simulink model "Manuf30_M8"  (R2023a)
settings: Solver=FixedStepAuto  StartTime=0.0  StopTime=720  FixedStep=1  RelTol=1e-3
model workspace (MAT data in the model file):
  EPdefault = 5
  EPmax = 5
  FRm = 120
  IPdefault = 5
libraries: simulink x25
(part 1 of 2)
settings Model: PacingRate=63  Creator=Boris Petrenj  LastModifiedBy=bramb
settings OptimizationCC: DefaultParameterBehavior=Inlined  EnhancedBackFolding=on  PassReuseOutputArgsAs=Individual arguments  ZeroExternalMemoryAtStartup=off  ZeroInternalMemoryAtStartup=off  OptimizeBlockOrder=speed  DifferentSizesBufferReuse=on  OptimizationCustomize=off  EfficientTunableParamExpr=on
settings DebuggingCC: ParameterTunabilityLossMsg=error  UnconnectedInputMsg=warning  UnconnectedOutputMsg=warning  UnconnectedLineMsg=warning  UnderSpecifiedDimensionMsg=warning
settings HardwareCC: TargetBitPerPointer=64  TargetBitPerSizeT=64  TargetBitPerPtrDiffT=64  TargetLongLongMode=on  TargetIntDivRoundTo=Zero  TargetEndianess=LittleEndian  TargetWordSize=64  TargetHWDeviceType=MATLAB Host  ProdEqTarget=off
settings ModelReferenceCC: EnableRefExpFcnMdlSchedulingChecks=on
settings SFSimCC: MATLABDynamicMemAlloc=off
settings RTWCC: Description=Embedded Coder  SystemTargetFile=ert.tlc  TemplateMakefile=ert_default_tmf  RTWVerbose=off  DLArmComputeVersion=19.05
settings CodeAppCC: ForceParamTrailComments=on  IgnoreCustomStorageClasses=off  OperatorAnnotations=on  SimulinkDataObjDesc=on  SFDataObjDesc=on  InsertBlockDesc=on
settings ERTTargetCC: GenerateSampleERTMain=on  SupportContinuousTime=on  InlinedParameterPlacement=NonHierarchical  ERTCustomFileTemplate=example_file_process.tlc

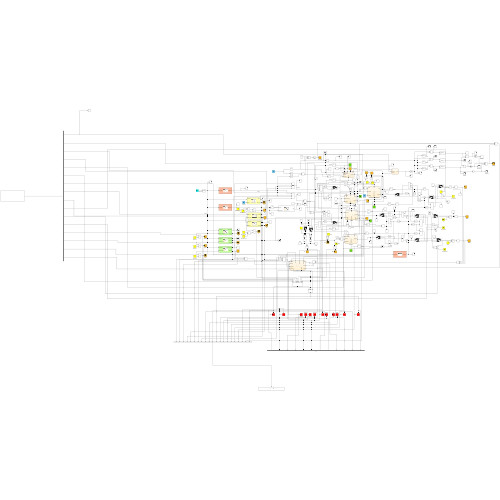
[thumbnail: Simulink's stored preview of the top-level diagram]
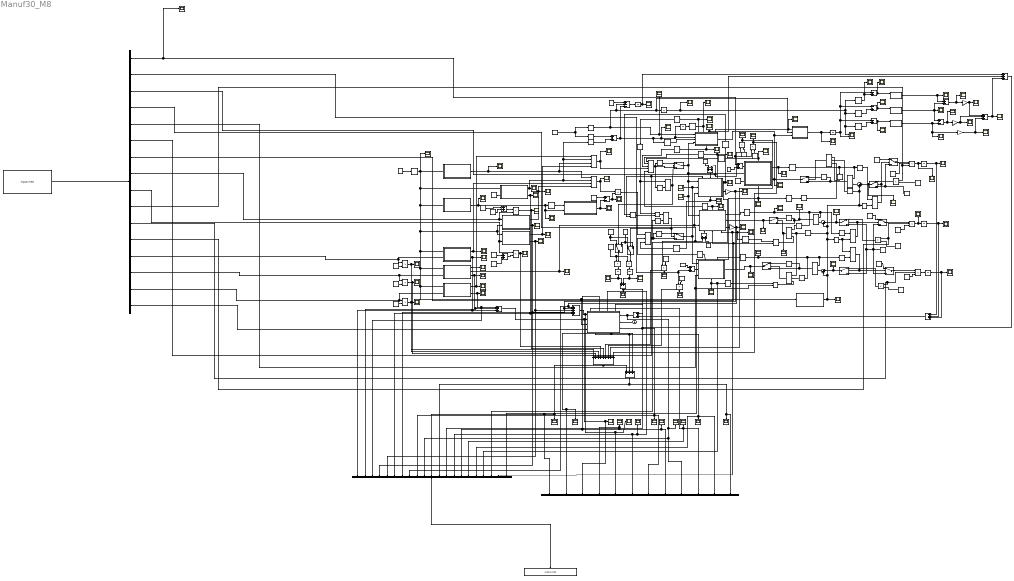
== system Manuf30_M8 ==
  AB : Scope
  AB deployment : Constant  Value=0.05
  ABackup price : Constant  Value=0.075
  AED : Scope
  Add : Sum  Inputs=+-
  Add{1,5..9,18..20} (9 alike) : Sum
  Add10 : Sum  Inputs=+-
  Add11 : Sum  Inputs=+-
  Add{12,14,16..17,22} (5 alike) : Sum  Inputs=+++
  Add13 : Sum  Inputs=+--
  Add15 : Sum  Inputs=+++++
  Add2 : Sum  Inputs=-+
  Add21 : Sum  Inputs=+++++++++
  Add3 : Sum  Inputs=-+
  Add4 : Sum  Inputs=-+
  BCI : Scope
  CancelledOrd : Scope
  Chart : Stateflow chart  TreatAsAtomicUnit=on
      settings: PortSchema="{\"entries\":[{\"content\":{\"sides\":[{\"content\":{\"connectorIds\":[\"In4\",\"In6\",\"In3\",\"In1\"]},\"type\":\"ConnectorPlacement.EquallySpacedRectSide\",\"uuid\":\"11f0d52a-88fc-4be5-bdc7-a55aa2612482\"},{\"content\":{\"connectorIds\":[\"In5\"],\"side\":\"RIGHT\"},\"type\":\"ConnectorPlacement.EquallySpacedRectSide\",\"uuid\":\"6f764515-397a-44dd-a2e9-3187fcbf9d3b\"},{\"content\":{\"connectorIds\":[\"Out3\",\"In2\",\"Out2\",\"In7\"],\"side\":\"TOP\"},\"type\":\"ConnectorPlacement.EquallySpacedRectSide\",\"uuid\":\"b2e58044-1c1f-45c5-a6c7-94a0948bfd55\"},{\"content\":{\"connectorIds\":[\"Out1\"],\"side\":\"BOTTOM\"},\"type\":\"ConnectorPlacement.EquallySpacedRectSide\",\"uuid\":\"446d024b-4857-45c6-b7aa-d3981b2b5c40\"}]},\"type\":\"ConnectorPlacement.EquallySpacedConnector\",\"uuid\":\"b78e99a1-1936-4240-9e27-63b28b547cdb\"}],\"packageUris\":[\"http://schema.mathworks.com/mf0/Connector/R2020b\"],\"version\":\"1.0\"}"
  Chart1 : Stateflow chart  TreatAsAtomicUnit=on
      settings: PortSchema="{\"entries\":[{\"content\":{\"sides\":[{\"content\":{\"connectorIds\":[\"In3\",\"In2\",\"In4\",\"In5\"]},\"type\":\"ConnectorPlacement.EquallySpacedRectSide\",\"uuid\":\"378523c1-40c5-4401-902f-aeb832ff0c9f\"},{\"content\":{\"connectorIds\":[\"In6\",\"In7\",\"In1\"],\"side\":\"RIGHT\"},\"type\":\"ConnectorPlacement.EquallySpacedRectSide\",\"uuid\":\"7940ff85-ee40-44d5-9690-9128d9333e88\"},{\"content\":{\"connectorIds\":[\"Out3\",\"Out5\",\"Out6\",\"Out4\"],\"side\":\"TOP\"},\"type\":\"ConnectorPlacement.EquallySpacedRectSide\",\"uuid\":\"ed54a4f9-7485-4487-a378-6fa31cb94842\"},{\"content\":{\"connectorIds\":[\"Out1\",\"Out2\"],\"side\":\"BOTTOM\"},\"type\":\"ConnectorPlacement.EquallySpacedRectSide\",\"uuid\":\"59aa636e-9062-4d7b-b9aa-b7c99c05c2d5\"}]},\"type\":\"ConnectorPlacement.EquallySpacedConnector\",\"uuid\":\"5563ec8e-56bc-49dd-8f68-3b08d3fc6c7f\"}],\"packageUris\":[\"http://schema.mathworks.com/mf0/Connector/R2020b\"],\"version\":\"1.0\"}"
  Chart2 : Stateflow chart  TreatAsAtomicUnit=on
      settings: PortSchema="{\"entries\":[{\"content\":{\"sides\":[{\"content\":{\"connectorIds\":[\"Out1\",\"In2\",\"In1\"]},\"type\":\"ConnectorPlacement.EquallySpacedRectSide\",\"uuid\":\"1d54177f-2d9d-4f9f-bcdb-576a16328a05\"},{\"content\":{\"connectorIds\":[\"Out2\"],\"side\":\"RIGHT\"},\"type\":\"ConnectorPlacement.EquallySpacedRectSide\",\"uuid\":\"203a6c5b-a59e-424a-95d4-58501034805f\"},{\"content\":{\"connectorIds\":[],\"side\":\"TOP\"},\"type\":\"ConnectorPlacement.EquallySpacedRectSide\",\"uuid\":\"eef511bd-9515-4db3-88d2-ce1a818e3fa2\"}]},\"type\":\"ConnectorPlacement.EquallySpacedConnector\",\"uuid\":\"79254a1d-868f-4542-aa12-bb7c48326cb6\"}],\"packageUris\":[\"http://schema.mathworks.com/mf0/Connector/R2020b\"],\"version\":\"1.0\"}"
  Clock : Clock
  Compare To Constant{,2..3,9} (4 alike) : simulink/Logic and Bit Operations/Compare To Constant  relop=>  const=0.9  OutDataTypeStr=boolean
  Compare To Constant1 : simulink/Logic and Bit Operations/Compare To Constant  relop=>  const=1  OutDataTypeStr=boolean
  Compare To Constant10 : simulink/Logic and Bit Operations/Compare To Constant  relop=>=  const=1.7  OutDataTypeStr=boolean
  Compare To Constant11 : simulink/Logic and Bit Operations/Compare To Constant  relop=>  const=1  OutDataTypeStr=boolean
  Compare To Constant12 : simulink/Logic and Bit Operations/Compare To Constant  relop=<  const=0.9  OutDataTypeStr=boolean
  Compare To Constant13 : simulink/Logic and Bit Operations/Compare To Constant  relop=>  const=0  OutDataTypeStr=boolean
  Compare To Constant4 : simulink/Logic and Bit Operations/Compare To Constant  relop=<  const=0.9  OutDataTypeStr=boolean
  Compare To Constant5 : simulink/Logic and Bit Operations/Compare To Constant  relop=>=  const=1.7  OutDataTypeStr=boolean
  Compare To Constant6 : simulink/Logic and Bit Operations/Compare To Constant  relop=>=  const=1.7  OutDataTypeStr=boolean
  Compare To Constant7 : simulink/Logic and Bit Operations/Compare To Constant  relop=>  const=0  OutDataTypeStr=boolean
  Compare To Constant8 : simulink/Logic and Bit Operations/Compare To Constant  relop=>  const=0  OutDataTypeStr=boolean
  Const : Constant  Value=0
  Const1 : Constant  Value=0
  Const{2..3,5..6} (4 alike) : Constant
  Const4 : Constant  Value=0
  Constant : Constant
  Constant11 : Constant  Value=8.5
  Constant2 : Constant
  Constant3 : Constant
  Delay : Delay  DelayLength=30  DelayLengthUpperLimit=5  InitialCondition=1  SampleTime=1
  Delay{1..3,5,7..8} (6 alike) : Delay  DelayLength=1  DelayLengthUpperLimit=5  InitialCondition=3  SampleTime=1
  Delay10 : Delay  DelayLength=1  DelayLengthUpperLimit=5  InitialCondition=IPdefault  SampleTime=1
  Delay{4,6,9,11..12,17} (6 alike) : Delay  DelayLength=1  DelayLengthUpperLimit=5  InitialCondition=1  SampleTime=1
  Delay13 : Delay  DelayLength=1  DelayLengthUpperLimit=5  InitialCondition=EPdefault  SampleTime=1
  Delay14 : Delay  DelayLength=60  DelayLengthUpperLimit=5  InitialCondition=0  SampleTime=1
  Delay15 : Delay  DelayLength=90  DelayLengthUpperLimit=5  InitialCondition=0  SampleTime=1
  Delay16 : Delay  DelayLength=30  DelayLengthUpperLimit=5  InitialCondition=0  SampleTime=1
  Delay18 : Delay  DelayLength=20  DelayLengthUpperLimit=5  InitialCondition=0.5  SampleTime=1
  Delay19 : Delay  DelayLength=100  DelayLengthUpperLimit=5  InitialCondition=0  SampleTime=1
  Delay20 : Delay  DelayLength=20  DelayLengthUpperLimit=5  InitialCondition=0  SampleTime=1
  Delay30 : Scope
  Delay60 : Scope
  Delay90 : Scope
  Demux : Demux  Outputs=16
  EP max : Constant  Value=10
  EPC : Constant  Value=0.01
  EPLoss : Scope
  EPS : Scope
  External : Stateflow chart  TreatAsAtomicUnit=on
      settings: PortSchema="{\"entries\":[{\"content\":{\"sides\":[{\"content\":{\"connectorIds\":[\"In1\",\"In4\"]},\"type\":\"ConnectorPlacement.EquallySpacedRectSide\",\"uuid\":\"f271faee-6a60-479d-a866-8a5439de7add\"},{\"content\":{\"connectorIds\":[\"Out1\",\"In5\",\"Out4\"],\"side\":\"RIGHT\"},\"type\":\"ConnectorPlacement.EquallySpacedRectSide\",\"uuid\":\"e4108372-e6fe-4c4b-a7e6-7abfa79efbb7\"},{\"content\":{\"connectorIds\":[\"Out2\"],\"side\":\"TOP\"},\"type\":\"ConnectorPlacement.EquallySpacedRectSide\",\"uuid\":\"57ee2673-3adc-41fc-b7cf-33ada2fd2761\"},{\"content\":{\"connectorIds\":[\"In2\",\"In3\",\"Out3\"],\"side\":\"BOTTOM\"},\"type\":\"ConnectorPlacement.EquallySpacedRectSide\",\"uuid\":\"ef56ac79-8641-40f7-a011-edb5fa111627\"}]},\"type\":\"ConnectorPlacement.EquallySpacedConnector\",\"uuid\":\"67aaf845-721f-4bae-9783-ff666cd7a7bd\"}],\"packageUris\":[\"http://schema.mathworks.com/mf0/Connector/R2020b\"],\"version\":\"1.0\"}"
  FINAL : Scope
  "FPC " : Constant  Value=0.012
  FPS : Scope
  FPdefault : Constant
  FPmax : Constant  Value=10
  Finished Products Warehouse : Stateflow chart  TreatAsAtomicUnit=on
      settings: PortSchema="{\"entries\":[{\"content\":{\"sides\":[{\"content\":{\"connectorIds\":[\"In3\",\"In2\",\"In1\"]},\"type\":\"ConnectorPlacement.EquallySpacedRectSide\",\"uuid\":\"a927ef52-d91a-4dcc-84e0-b91b0cab93cc\"},{\"content\":{\"connectorIds\":[\"Out2\",\"In4\"],\"side\":\"RIGHT\"},\"type\":\"ConnectorPlacement.EquallySpacedRectSide\",\"uuid\":\"3748cd02-f2f9-44a2-8c75-23a4abadb7cf\"},{\"content\":{\"connectorIds\":[\"Out1\"],\"side\":\"TOP\"},\"type\":\"ConnectorPlacement.EquallySpacedRectSide\",\"uuid\":\"31dbc187-02a7-4af9-af69-01f7c7d572fd\"},{\"content\":{\"connectorIds\":[\"Out3\"],\"side\":\"BOTTOM\"},\"type\":\"ConnectorPlacement.EquallySpacedRectSide\",\"uuid\":\"61372254-f33a-42e5-a460-357783406dca\"}]},\"type\":\"ConnectorPlacement.EquallySpacedConnector\",\"uuid\":\"01135270-3585-4456-b5cd-d6a08ddd9ae5\"}],\"packageUris\":[\"http://schema.mathworks.com/mf0/Connector/R2020b\"],\"version\":\"1.0\"}"
  From File : FromFile  FileName=input.mat  SampleTime=0
  Gain : Gain  Gain=0.8
  Gain1 : Gain  Gain=0.5
  Gain2 : Gain  Gain=0.2
  Gain4 : Gain  Gain=0.2
  Gain5 : Gain  Gain=0.4
  IPC : Constant  Value=0.01
  IPLoss : Scope
  IPS : Scope
  IPmax : Constant  Value=10
  IT backup : Constant  Value=0
  ITC : Constant  Value=0.002
  ITC1 : Constant  Value=0.002
  ITD : Scope
  InEPC : Scope
  InRMC : Scope
  Integrator{,1..8} (9 alike) : Integrator  ZeroCross=off
  Internal : Stateflow chart  TreatAsAtomicUnit=on
      settings: PortSchema="{\"entries\":[{\"content\":{\"sides\":[{\"content\":{\"connectorIds\":[\"In1\",\"In4\",\"In5\"]},\"type\":\"ConnectorPlacement.EquallySpacedRectSide\",\"uuid\":\"bafe3ab1-f241-4393-bddb-ef475e1fdd49\"},{\"content\":{\"connectorIds\":[\"Out4\",\"Out1\"],\"side\":\"RIGHT\"},\"type\":\"ConnectorPlacement.EquallySpacedRectSide\",\"uuid\":\"094e9ebe-ff1f-4efe-a044-3eef12cc294d\"},{\"content\":{\"connectorIds\":[\"In3\",\"In2\",\"Out2\"],\"side\":\"TOP\"},\"type\":\"ConnectorPlacement.EquallySpacedRectSide\",\"uuid\":\"3b7b6677-6a8b-48f7-ba0f-1ece0b251949\"},{\"content\":{\"connectorIds\":[\"Out3\"],\"side\":\"BOTTOM\"},\"type\":\"ConnectorPlacement.EquallySpacedRectSide\",\"uuid\":\"83286e05-32a8-4169-bad3-c8b6d6ae35ee\"}]},\"type\":\"ConnectorPlacement.EquallySpacedConnector\",\"uuid\":\"adc1cee4-8036-4ca5-bb72-3dad1999a28e\"}],\"packageUris\":[\"http://schema.mathworks.com/mf0/Connector/R2020b\"],\"version\":\"1.0\"}"
  LBC : Scope
  LBuilding : Scope
  LCD : Scope
  LCR price : Constant  Value=0.05
  LCRC : Scope
  LProfit : Scope
  LProperty : Scope
  Logical Operator{,1,4..5,7} (5 alike) : Logic  AllPortsSameDT=off  OutDataTypeStr=boolean
  Logical Operator2 : Logic  Inputs=3  AllPortsSameDT=off  OutDataTypeStr=boolean
  Logical Operator3 : Logic  Inputs=3  AllPortsSameDT=off  OutDataTypeStr=boolean
  Logical Operator6 : Logic  Inputs=3  AllPortsSameDT=off  OutDataTypeStr=boolean
  Logical Operator8 : Logic  Operator=OR  AllPortsSameDT=off  OutDataTypeStr=boolean
  MB : Scope
  MB deployment : Constant  Value=0.05
  MBackup price : Constant  Value=0.125
  MED : Scope
  MFD : Scope
  MFR price : Constant  Value=0.09
  MFRC : Scope
  MinMax : MinMax  Inputs=4
  MinMax Running Resettable : simulink/Math Operations/MinMax Running Resettable  Function=max  vinit=0.0
  MinMax Running Resettable1 : simulink/Math Operations/MinMax Running Resettable  Function=max  vinit=0.0
  MinMax Running Resettable2 : simulink/Math Operations/MinMax Running Resettable  Function=max  vinit=0.0
  MinMax1 : MinMax  Inputs=4
  MinMax2 : MinMax  Inputs=5
  MinMax3 : MinMax  Inputs=3
  MinMax4 : MinMax  Inputs=2
  MinMax5 : MinMax  Inputs=2
  MinMax6 : MinMax  Inputs=2
  MissedSales : Scope
  Mux : Mux  Inputs=12
  Mux1 : Mux  Inputs=21
  NLBC : Scope
  NLBuilding : Scope
  NLProfit : Scope
  NLProperty : Scope
  NetLoss : Scope
  OTC : Constant  Value=0.003
  OVT : Scope
  OVTA : Scope
  OVTM : Scope
  OutC : Scope
  Overtime daily : Constant  Value=0.005
  Penalty{,30,60,90} (4 alike) : Scope
  Premium : Scope
  Product{,1..2,5..13,15..17} (15 alike) : Product
  Product14 : Product  Inputs=3
  Product3 : Product  Inputs=3
  Product4 : Product  Inputs=3
  RM max : Constant  Value=20
  RMC : Constant  Value=0.004
  RMS : Scope
  Raw Material : Stateflow chart  TreatAsAtomicUnit=on
      settings: PortSchema="{\"entries\":[{\"content\":{\"sides\":[{\"content\":{\"connectorIds\":[\"In4\",\"In3\",\"In2\"]},\"type\":\"ConnectorPlacement.EquallySpacedRectSide\",\"uuid\":\"22025498-79bd-4643-822c-161eb7d47779\"},{\"content\":{\"connectorIds\":[\"In1\"],\"side\":\"RIGHT\"},\"type\":\"ConnectorPlacement.EquallySpacedRectSide\",\"uuid\":\"aa922f6c-a4fe-4fc7-972b-8ab2307e949a\"},{\"content\":{\"connectorIds\":[\"Out1\",\"Out2\"],\"side\":\"TOP\"},\"type\":\"ConnectorPlacement.EquallySpacedRectSide\",\"uuid\":\"c86c8a9f-a244-4d8b-968a-c1875225a868\"},{\"content\":{\"connectorIds\":[\"Out3\"],\"side\":\"BOTTOM\"},\"type\":\"ConnectorPlacement.EquallySpacedRectSide\",\"uuid\":\"eeeb2d52-6864-42d6-8395-63d54164c7a9\"}]},\"type\":\"ConnectorPlacement.EquallySpacedConnector\",\"uuid\":\"5943e233-3d2e-4fc1-b9ec-0b2299862940\"}],\"packageUris\":[\"http://schema.mathworks.com/mf0/Connector/R2020b\"],\"version\":\"1.0\"}"
  Relational Operator : RelationalOperator  Operator=<  OutDataTypeStr=boolean  RndMeth=Simplest  InputSameDT=off
  Relational Operator1 : RelationalOperator  Operator=<=  OutDataTypeStr=boolean  RndMeth=Simplest  InputSameDT=off
  Relational Operator2 : RelationalOperator  Operator=<  OutDataTypeStr=boolean  RndMeth=Simplest  InputSameDT=off
  Scope{,1..25,27,29,31..34,36..53,55,57,61..62} (54 alike) : Scope
  Scope30 : Scope  NumInputPorts=2
  Slider Gain : simulink/Math Operations/Slider Gain  gain=0.250  low=0  high=1
  Slider Gain1 : simulink/Math Operations/Slider Gain  gain=0.250  low=0  high=1
  Slider Gain2 : simulink/Math Operations/Slider Gain  gain=0.500  low=0  high=1
  Slider Gain{3..7} (5 alike) : simulink/Math Operations/Slider Gain  gain=1.75  low=1  high=2
  State Transition Table : State Transition Table  TreatAsAtomicUnit=on
  State Transition Table1 : State Transition Table  TreatAsAtomicUnit=on
  State Transition Table2 : State Transition Table  TreatAsAtomicUnit=on
  State Transition Table3 : State Transition Table  TreatAsAtomicUnit=on
  State Transition Table4 : State Transition Table  TreatAsAtomicUnit=on
  State Transition Table5 : State Transition Table  TreatAsAtomicUnit=on
  State Transition Table6 : State Transition Table  TreatAsAtomicUnit=on
  State Transition Table7 : State Transition Table  TreatAsAtomicUnit=on
      settings: PortSchema="{\"entries\":[{\"content\":{\"sides\":[{\"content\":{\"connectorIds\":[\"In2\",\"In1\"]},\"type\":\"ConnectorPlacement.EquallySpacedRectSide\",\"uuid\":\"973c4974-d7c3-495b-af66-41138f62d073\"},{\"content\":{\"connectorIds\":[\"Out1\",\"Out2\"],\"side\":\"RIGHT\"},\"type\":\"ConnectorPlacement.EquallySpacedRectSide\",\"uuid\":\"88ce3e21-147c-464e-840e-98ee58d70a4b\"},{\"content\":{\"connectorIds\":[],\"side\":\"TOP\"},\"type\":\"ConnectorPlacement.EquallySpacedRectSide\",\"uuid\":\"4640dcaa-34f7-4581-b763-3c6a5a253cb1\"}]},\"type\":\"ConnectorPlacement.EquallySpacedConnector\",\"uuid\":\"d1b0acb9-137d-4050-9d83-c9297b746b08\"}],\"packageUris\":[\"http://schema.mathworks.com/mf0/Connector/R2020b\"],\"version\":\"1.0\"}"
  State Transition Table8 : State Transition Table  TreatAsAtomicUnit=on
  State Transition Table9 : State Transition Table  TreatAsAtomicUnit=on
  Sum1 : Sum  Inputs=|++
  Sum2 : Sum  Inputs=|++
  Sum3 : Sum  Inputs=|++
  Switch{,1..11,13} (13 alike) : Switch  Criteria=u2 > Threshold  Threshold=0.5  SaturateOnIntegerOverflow=off  InputSameDT=off
  To File : ToFile  Filename=output.mat
  Truck capacity : Constant  Value=0.03
  Truck capacity1 : Constant  Value=0.04
  Truck capacity2 : Constant  Value=0.05
  WD : Scope
  WR price : Constant  Value=0.05
  WRC : Scope
  wires:
  State Transition Table2/1(Electricity) -> MinMax1/3, MinMax/1, Scope39/1  "Electricity"
  State Transition Table9/1(ITEq) -> Scope41/1, Slider Gain/1, MinMax1/2, MinMax/2  "IT system"
  Add/1 -> Scope20/1, Product/2
  Delay/1 -> State Transition Table/1(Delayed)  "Delayed"
  State Transition Table/1(Mnf) -> Scope/1, Add/2
  MinMax/1 -> Scope1/1, Product/1
  Constant/1 -> Add/1
  Product/1 -> MinMax3/1  "Manufacturing"
  Internal/4(IParts) -> Mux1/19, Delay10/1, Scope4/1
  MinMax1/1 -> MinMax2/4, Scope18/1  "Assembly"
  State Transition Table3/1(Maintenance) -> Scope21/1, State Transition Table/2(Maintenance), Delay/1, Scope29/1
  Switch/1 -> Raw Material/4(Manufacturing), Scope44/1, Internal/4(Manufacturing)
  Raw Material/2(LxRM) -> Delay5/1
  Delay1/1 -> MinMax2/2  "Delayed"
  Delay2/1 -> MinMax3/3  "Delayed"
  Delay3/1 -> MinMax3/2  "Delayed"
  Raw Material/1(MxRM) -> Delay3/1
  Internal/2(AxIP) -> Delay1/1, Scope5/1
  External/1(LxEP) -> Delay4/1
  Delay4/1 -> Compare To Constant5/1, Compare To Constant7/1, MinMax4/1, Scope12/1  "Delayed"
  Delay5/1 -> Scope47/1, Compare To Constant6/1, MinMax6/1, Compare To Constant8/1  "Delayed"
  MinMax4/1 -> Slider Gain5/1, Switch3/3, Scope31/1  "Inbound Logistics"
  External/2(AxEP) -> Delay6/1, Scope10/1
  Delay6/1 -> MinMax2/5  "Delayed"
  Finished Products Warehouse/3(FinishedProducts) -> Delay17/1, Mux1/21, Scope13/1
  Delay8/1 -> MinMax2/1  "Delayed"
  Chart/1(AxO) -> Scope15/1, Delay9/1
  Delay9/1 -> MinMax2/3  "Delayed"
  Finished Products Warehouse/2(LxFP) -> Scope16/1, Delay7/1
  Delay7/1 -> Compare To Constant13/1, MinMax5/1, Compare To Constant10/1  "Delayed"
  Constant3/1 -> Slider Gain2/1, Slider Gain1/1
  Demux/10 -> Product1/1, Product4/3
  Truck capacity/1 -> Product1/2
  Slider Gain/1 -> Add1/2
  Slider Gain1/1 -> Add1/1
  Slider Gain2/1 -> Scope45/1, Chart/4(Contracts), Add13/2, Chart2/2(Contracts), Integrator1/1
  Chart/3(Orders) -> Delay11/1, Scope14/1
  Demux/12 -> Product3/2, Product2/1
  Truck capacity1/1 -> Product2/2
  Constant11/1 -> Delay19/1  "Magnitude"
  Delay16/1 -> Scope23/1, Add2/2  "Delayed"
  Add2/1 -> MinMax Running Resettable/1, Scope34/1
  Delay14/1 -> Add3/2  "Delayed"
  Delay15/1 -> Add4/2  "Delayed"
  Add3/1 -> Scope32/1, MinMax Running Resettable1/1
  Add4/1 -> MinMax Running Resettable2/1, Scope22/1
  State Transition Table1/1(MainFacility) -> Scope37/1, MinMax/3
  State Transition Table5/1(Warehouse) -> Scope38/1
  State Transition Table6/1(LogisticsCenter) -> Scope40/1, MinMax1/1
  State Transition Table8/1(AssemEq) -> Scope43/1, MinMax1/4
  State Transition Table7/1(ManufEq) -> Scope42/1, MinMax/4
  Demux/5 -> Raw Material/2(RMdefault), Relational Operator1/2
  Demux/6 -> Internal/3(IPdefault), Relational Operator/2
  Finished Products Warehouse/1(AxFP) -> Delay8/1, Scope17/1
  FPdefault/1 -> Finished Products Warehouse/1(FPdefault)
  Demux/7 -> External/3(EPdefault), Relational Operator2/2
  External/3(EParts) -> Mux1/20, Delay13/1, Scope8/1
  External/4(Loss) -> Gain4/1
  Switch1/1 -> Chart/1(Assembly), External/1(Assembly), Scope2/1, Internal/1(Assembly), Finished Products Warehouse/2(Assembly)
  Internal/1(LossIP) -> Gain5/1
  Delay11/1 -> Compare To Constant1/1  "Delayed"
  Compare To Constant1/1 -> Logical Operator8/1, Logical Operator1/1
  Relational Operator/1 -> Logical Operator8/2
  Delay10/1 -> Relational Operator/1  "Delayed"
  MinMax3/1 -> Compare To Constant/1, Switch/3, Slider Gain3/1
  Slider Gain3/1 -> Switch/1
  Compare To Constant/1 -> Logical Operator/2
  Logical Operator/1 -> Switch11/2, Switch/2
  MinMax2/1 -> Compare To Constant2/1, Slider Gain4/1, Switch1/3
  Slider Gain4/1 -> Switch1/1
  Logical Operator1/1 -> Switch10/2, Switch1/2
  Compare To Constant2/1 -> Logical Operator1/2
  Product2/1 -> Switch4/1
  Switch4/1 -> Sum1/1, Scope7/1
  Raw Material/3(RawMaterial) -> Mux1/18, Delay12/1, Scope3/1
  Relational Operator1/1 -> Logical Operator3/3
  Relational Operator2/1 -> Logical Operator2/3
  Compare To Constant3/1 -> Logical Operator3/1, Logical Operator2/2
  Switch3/1 -> External/5(Logistics), Scope11/1
  Slider Gain5/1 -> Switch3/1
  Logical Operator2/1 -> Scope33/1, Switch3/2
  Compare To Constant4/1 -> Logical Operator5/1, Logical Operator4/2
  Compare To Constant5/1 -> Logical Operator2/1
  Delay12/1 -> Relational Operator1/1  "Delayed"
  Delay13/1 -> Relational Operator2/1  "Delayed"
  Internal/3(MxIP) -> Scope6/1, Delay2/1
  Switch5/1 -> Scope46/1, Raw Material/1(Logistics)
  Slider Gain6/1 -> Switch5/1
  Compare To Constant6/1 -> Logical Operator3/2
  MinMax6/1 -> Slider Gain6/1, Switch5/3  "Inbound Logistics"
  Logical Operator3/1 -> Switch5/2
  Const/1 -> Switch13/3, Switch4/3, Switch6/3, Switch8/3
  Compare To Constant7/1 -> Logical Operator4/1
  Logical Operator4/1 -> Switch8/2, Switch4/2
  State Transition Table4/1(Logistics) -> Sum3/2, Compare To Constant4/1, Compare To Constant3/1, Sum1/2, Compare To Constant9/1, Sum2/2, Compare To Constant12/1, Scope9/1
  Sum1/1 -> MinMax4/2
  Compare To Constant8/1 -> Logical Operator5/2
  Logical Operator5/1 -> Switch13/2, Switch6/2
  Switch6/1 -> Scope27/1, Sum3/1
  Sum3/1 -> MinMax6/2
  Product1/1 -> Switch2/1
  Const1/1 -> Switch9/3, Switch2/3
  Sum2/1 -> MinMax5/2
  Switch2/1 -> Sum2/1, Scope48/1
  Logical Operator6/1 -> Switch7/2
  MinMax5/1 -> Switch7/3, Slider Gain7/1
  Slider Gain7/1 -> Switch7/1
  Compare To Constant9/1 -> Logical Operator6/2
  Compare To Constant10/1 -> Logical Operator6/1
  Delay17/1 -> Compare To Constant11/1  "Delayed"
  Compare To Constant11/1 -> Logical Operator6/3
  Compare To Constant12/1 -> Logical Operator7/2
  Compare To Constant13/1 -> Logical Operator7/1
  Logical Operator7/1 -> Switch9/2, Switch2/2
  Const2/1 -> Switch8/1
  Switch8/1 -> Product3/1
  ITC/1 -> Product3/3
  Product3/1 -> Scope51/1, Integrator2/1
  Integrator2/1 -> Add17/2, InEPC/1
  Const3/1 -> Switch9/1
  Switch9/1 -> Product4/1
  OTC/1 -> Product4/2
  Product4/1 -> Scope53/1, Integrator3/1
  Integrator3/1 -> Add17/1, OutC/1
  Add5/1 -> Finished Products Warehouse/3(FPmax)
  Demux/1 -> Scope25/1, Add5/1, Product5/1
  FPmax/1 -> Add5/2
  Product5/1 -> Add21/9, FPS/1
  "FPC "/1 -> Product5/2
  Add6/1 -> Internal/2(IPmax)
  IPmax/1 -> Add6/1
  Demux/3 -> Add6/2, Product6/1
  IPC/1 -> Product6/2
  Product6/1 -> Add21/8, IPS/1
  Add7/1 -> External/2(EPmax)
  Demux/4 -> Add7/1, Product7/1
  EP max/1 -> Add7/2
  Product7/1 -> Add21/6, EPS/1
  EPC/1 -> Product7/2
  Add8/1 -> Raw Material/3(RMmax)
  RM max/1 -> Add8/1
  Demux/2 -> Add8/2, Product8/1
  RMC/1 -> Product8/2
  Product8/1 -> Add21/7, RMS/1
  Demux/9 -> Product9/1, State Transition Table8/2(Backup)
  Demux/8 -> Product10/2, State Transition Table7/2(Backup)
  Product9/1 -> Add21/4, AB/1
  Product10/1 -> Add21/5, MB/1
  Switch10/1 -> Product11/2
  Product11/1 -> Integrator4/1
  Integrator4/1 -> OVTA/1, Add9/1
  Const5/1 -> Switch11/1, Switch10/1
  Const4/1 -> Switch11/3, Switch10/3
  Switch11/1 -> Product12/2
  Overtime daily/1 -> Product12/1, Product11/1
  Product12/1 -> Integrator5/1
  Integrator5/1 -> Add9/2, OVTM/1
  Add9/1 -> Add18/1, OVT/1
  Logical Operator8/1 -> Logical Operator/1
  Add10/1 -> Delay60/1, Gain1/1
  Add11/1 -> Gain2/1, Delay30/1
  Gain/1 -> Add12/3, Penalty90/1
  Gain1/1 -> Add12/2, Penalty60/1
  Gain2/1 -> Add12/1, Penalty30/1
  Add12/1 -> Add16/3, Penalty/1
  Constant2/1 -> Add13/1
  IT backup/1 -> State Transition Table9/2(Backup)
  Add13/1 -> Integrator6/1
  Integrator6/1 -> Add16/1, MissedSales/1
  Delay19/1 -> Scope50/1, State Transition Table9/1(Magnitude), State Transition Table4/1(Magnitude), Chart1/4(Magnitude), State Transition Table6/1(Magnitude), State Transition Table5/1(Magnitude), State Transition Table1/1(Magnitude), State Transition Table8/1(Magnitude), State Transition Table7/1(Magnitude), State Transition Table3/1(Magnitude), State Transition Table2/1(Magnitude)  "Delayed"
  Add1/1 -> Add13/3, Delay18/1, Scope24/1, Integrator8/1, Chart/6(MarketingSales)
  MinMax Running Resettable1/1 -> Add11/2, Scope36/1, Add10/1
  MinMax Running Resettable2/1 -> Add10/2, Delay90/1, Gain/1
  Integrator1/1 -> Scope57/1, Scope30/1, Delay15/1, Delay14/1, Delay16/1
  Integrator8/1 -> Delay20/1
  Delay20/1 -> Chart/2(Sold), Scope55/1  "Delayed"
  Switch7/1 -> Chart/5(Logistics), Chart2/1(Logistics), Scope19/1, Finished Products Warehouse/4(Logistics)
  Integrator/1 -> Scope30/2, Add2/1, Add3/1, Add4/1
  MinMax Running Resettable/1 -> Scope52/1, Add11/1
  Gain4/1 -> EPLoss/1, Mux1/8, Add15/1
  Gain5/1 -> IPLoss/1, Mux1/7, Add15/2
  Delay18/1 -> Chart/3(MSdelay)  "Delayed"
  Const6/1 -> Switch13/1
  Demux/11 -> Product14/2, Product13/1
  Product14/1 -> Integrator7/1
  Integrator7/1 -> Add17/3, InRMC/1
  ITC1/1 -> Product14/3
  Switch13/1 -> Product14/1
  Truck capacity2/1 -> Product13/2
  Product13/1 -> Switch6/1
  State Transition Table1/2(Damage) -> Mux1/1, Add14/3, MFD/1
  State Transition Table5/3(Damage) -> Mux1/2, Add14/2, WD/1
  State Transition Table6/2(Damage) -> Mux1/3, Add14/1, LCD/1
  State Transition Table7/2(Damage) -> Mux1/4, Add15/4, MED/1
  State Transition Table9/2(Damage) -> Mux1/6, Add15/5, ITD/1
  State Transition Table8/2(Damage) -> Mux1/5, Add15/3, AED/1
  Chart/2(Loss) -> Add16/2, CancelledOrd/1
  Add17/1 -> Add18/2
  Add15/1 -> LProperty/1, Mux/5, Chart1/3(LProperty)
  Add14/1 -> LBuilding/1, Mux/3, Chart1/2(LBuilding)
  Demux/16 -> Chart1/5(Insurance)
  Add18/1 -> Mux/9, Mux1/10, LBC/1, Chart1/6(LBC)
  Add16/1 -> Mux/7, LProfit/1, Mux1/9, Chart1/1(LProfit)
  Chart1/1(NL) -> Add22/2, Mux1/17, Mux/11, NetLoss/1
  Clock/1 -> Chart1/7(Clock)
  Chart1/2(Premium) -> Mux/2, Premium/1, Add22/3
  Chart2/1(CR) -> Chart/7(CR), Scope61/1
  Chart2/2(Level) -> Scope62/1, Integrator/1
  Demux/13 -> State Transition Table1/2(Reinforcement), Product15/1
  Demux/15 -> State Transition Table6/2(Reinforcement), Product17/1
  Demux/14 -> State Transition Table5/2(Reinforcement), Product16/1
  MFR price/1 -> Product15/2
  WR price/1 -> Product16/2
  LCR price/1 -> Product17/2
  Product15/1 -> Add21/3, MFRC/1
  Product16/1 -> Add21/2, WRC/1
  Product17/1 -> LCRC/1, Add21/1
  State Transition Table5/2(Inventory) -> Scope49/1, Internal/5(Inventory), External/4(Inventory)
  AB deployment/1 -> Add19/2
  ABackup price/1 -> Add19/1
  Add19/1 -> Product9/2
  Add20/1 -> Product10/1
  MBackup price/1 -> Add20/1
  MB deployment/1 -> Add20/2
  Add21/1 -> Add22/1, Mux/1, Mux1/11, BCI/1
  Chart1/3(NLBC) -> Mux1/16, Mux/10, NLBC/1
  Chart1/5(NLProfit) -> Mux1/15, NLProfit/1, Mux/8
  Chart1/6(NLProperty) -> Mux/6, Mux1/14, NLProperty/1
  Chart1/4(NLBuilding) -> Mux1/13, Mux/4, NLBuilding/1
  Add22/1 -> Mux1/12, Mux/12, FINAL/1
  From File/1 -> Demux/1
  Mux1/1 -> To File/1

== stateflow chart Manuf30_M8/State Transition Table7 ==
  state Init
    T=0;
    ManufEq=1;
    Damage=0;
  state Great
    ManufEq=0;
    RT=180;
    T=T+1;
  state Major
    ManufEq=0;
    RT=30;
    T=T+1;
  state Strong
    ManufEq=0
    RT=7;
    T=T+1;
  state Moderate
    ManufEq=0;
    RT=1;
    T=T+1;
  state MBackup
    ManufEq=0;
    RT=5;
    T=T+1;
  state Over
    ManufEq=1;
  (default) -> Init
  Init -> (junction 29) [order 2] : [Magnitude>=7]
      | {Damage=5}
  (junction 29) -> (junction 23)
  Init -> (junction 41) [order 3] : [Magnitude>=6]
      | {Damage=2}
  (junction 41) -> (junction 39)
  Init -> (junction 44) [order 4] : [Magnitude>=5]
      | {Damage=0.5}
  (junction 44) -> (junction 32)
  Init -> Great [order 1] : [Magnitude>=8]
      | {Damage=10}
  Great -> (junction 134) [order 1] : [T>=RT]
      | {}
  (junction 134) -> (junction 137)
  Great -> (junction 156) [order 2] : [Backup>0]
  (junction 156) -> (junction 159)
  (junction 23) -> Major
  Major -> (junction 137) [order 1] : [T>=RT]
  (junction 137) -> (junction 140)
  Major -> (junction 159) [order 2] : [Backup>0]
  (junction 159) -> (junction 162)
  (junction 39) -> Strong
  Strong -> (junction 140) [order 1] : [T>=RT]
  (junction 140) -> (junction 143)
  Strong -> (junction 162) [order 2] : [Backup>0]
  (junction 162) -> (junction 154)
  (junction 32) -> Moderate
  Moderate -> (junction 143)
  (junction 143) -> (junction 132)
  (junction 154) -> MBackup
  MBackup -> Over : [T>=RT]
  (junction 132) -> Over
  data: Magnitude input; T local; RT local; ManufEq output; Backup input; Damage output

== stateflow chart Manuf30_M8/State Transition Table8 ==
  state Init
    T=0;
    AssemEq=1;
    Damage=0;
  state Great
    AssemEq=0;
    RT=180;
    T=T+1;
  state Major
    AssemEq=0;
    RT=20;
    T=T+1;
  state Strong
    AssemEq=0
    RT=7;
    T=T+1;
  state Moderate
    AssemEq=0;
    RT=1;
    T=T+1;
  state ABackup
    AssemEq=0;
    RT=4;
    T=T+1;
  state Over
    AssemEq=1;
  (default) -> Init
  Init -> (junction 29) [order 2] : [Magnitude>=7]
      | {Damage=2.5}
  (junction 29) -> (junction 23)
  Init -> (junction 41) [order 3] : [Magnitude>=6]
      | {Damage=1}
  (junction 41) -> (junction 39)
  Init -> (junction 44) [order 4] : [Magnitude>=5]
      | {Damage=0.25}
  (junction 44) -> (junction 32)
  Init -> Great [order 1] : [Magnitude>=8]
      | {Damage=5}
  Great -> (junction 134) [order 1] : [T>=RT]
  (junction 134) -> (junction 137)
  Great -> (junction 154) [order 2] : [Backup>0]
  (junction 154) -> (junction 157)
  (junction 23) -> Major
  Major -> (junction 137) [order 1] : [T>=RT]
  (junction 137) -> (junction 140)
  Major -> (junction 157) [order 2] : [Backup>0]
  (junction 157) -> (junction 160)
  (junction 39) -> Strong
  Strong -> (junction 140) [order 1] : [T>=RT]
  (junction 140) -> (junction 143)
  Strong -> (junction 160) [order 2] : [Backup>0]
  (junction 160) -> (junction 152)
  (junction 32) -> Moderate
  Moderate -> (junction 143)
  (junction 143) -> (junction 132)
  (junction 152) -> ABackup
  ABackup -> Over : [T>=RT]
  (junction 132) -> Over
  data: Magnitude input; T local; RT local; AssemEq output; Backup input; Damage output

== stateflow chart Manuf30_M8/External ==
  state Init
    EParts=EPdefault;
    LxEP=3;
    AxEP=3;
    Damage=0;
  state Update
    LxEP=3;
    AxEP=3;
    if (Inventory<1 && Damage==0)
    Loss=EParts*(1-Inventory);
    EParts=EParts*Inventory;
    Damage=1;
    end
    EParts = EParts + Logistics - Assembly;
    if EParts < 0
    AxEP=Logistics;
    EParts = 0;
    else if EParts > EPmax
    LxEP=Assembly;
    EParts = EPmax;
    end
    end
  state Full
    LxEP=Assembly;
    if Logistics >= Assembly
    EParts=EPmax;
    else
    EParts = EPmax + Logistics - Assembly
    end
  state Empty
    AxEP=Logistics;
    if Assembly>=Logistics
    EParts=0;
    else
    EParts= Logistics - Assembly;
    end
  (default) -> Init
  Init -> Update : [Assembly>0||Logistics>0||Inventory<1]
  Update -> Full [order 1] : [EParts>=EPmax]
  Full -> Update : [EParts<EPmax]
  Update -> Empty [order 2] : [EParts<=0]
  Empty -> Update : [EParts>0]
  data: Assembly input; EPmax input; EPdefault input; Inventory input; Logistics input; LxEP output; AxEP output; EParts output; Damage local; Loss output

== stateflow chart Manuf30_M8/Chart ==
  state Init
    AxO=3;
    Orders=1;
    OSales=0.5;
    ShippingS=0.5;
    ShippingC=0.5;
    ShippedS=0.5;
    Loss=0;
  state Update
    Orders = Orders + MarketingSales + Contracts - Assembly;
    AxO=3;
    ShippingS=0.5;
    ShippingC=0.5;
    ShippedS = ShippedS + ShippingS;
    if Orders < 0
    AxO=MarketingSales + Contracts;
    Orders = 0;
    end
    OSales = OSales + MarketingSales - ShippingS;
  state Empty
    AxO=MarketingSales + Contracts;
    if Assembly>=(MarketingSales+Contracts)
    Orders=0;
    else
    Orders= MarketingSales + Contracts - Assembly;
    end
  state ContractRecovery
    ShippingS=0;
    ShippingC=Logistics;
    Orders = Orders + MarketingSales + Contracts - Assembly;
    OSales = OSales + MarketingSales;
    if (Sold-ShippedS>0)
    Loss = Loss + MSdelay;
    Orders = Orders - MSdelay;
    OSales = OSales - MSdelay;
    end
  state SalesRecovery
    Orders = Orders + MarketingSales + Contracts - Assembly;
    if Logistics>=0,5
    ShippingC=0.5;
    ShippingS=Logistics-ShippingC;
    end
    if Logistics<0.5
    ShippingC=Logistics;
    ShippingS=0;
    end
    ShippedS = ShippedS + ShippingS;
    OSales = OSales + MarketingSales - ShippingS;
  (default) -> Init
  Update -> Empty [order 3] : [Orders<=0]
  Init -> Update : [MarketingSales>0||Assembly>0||Contracts>0]
  Empty -> Update : [Orders>0]
  SalesRecovery -> Update [order 2] : [OSales<=0.5]
  Update -> SalesRecovery [order 2] : [CR==0&OSales>0.5]
  Update -> ContractRecovery [order 1] : [CR]
  ContractRecovery -> Update [order 1] : [CR==0&OSales<=0.5]
  SalesRecovery -> ContractRecovery [order 1] : [CR]
  ContractRecovery -> SalesRecovery [order 2] : [CR==0&OSales>0.5]
  data: Assembly input; Sold input; MSdelay input; Contracts input; Logistics input; MarketingSales input; AxO output; Loss output; OSales local; ShippedS local; Orders output; ShippingS local; ShippingC local; CR input

== stateflow chart Manuf30_M8/Chart1 ==
  state Package1
    Premium=0.01;
    if LBuilding>10
    NLBuilding=LBuilding-10;
    else
    NLBuilding=0;
    end
    NLProperty=LProperty;
    NLProfit=LProfit;
    NLBC=LBC;
    NL=NLBuilding+NLProperty+NLProfit+NLBC;
  state Full
    Premium=0.15;
    Total=LBuilding+LProperty+LProfit;
    if Total>50
    CombinedLoss=Total-50;
    else
    CombinedLoss=0;
    end
    if Magnitude>8
    Coverage=20;
    end
    if Magnitude>7
    Coverage=15;
    end
    if Magnitude>6
    Coverage=10;
    end
    if Magnitude>5
    Coverage=7;
    end
    if LBC>Coverage
    NLBC=LBC-Coverage;
    else
    NLBC=0;
    end
    NL=CombinedLoss+NLBC;
  state NoInsurance
    NLBuilding=LBuilding;
    NLProperty=LProperty;
    NLProfit=LProfit;
    NLBC=LBC;
    NL=NLBuilding+NLProperty+NLProfit+NLBC;
  state Package2
    Premium=0.1;
    if LBuilding>10
    NLBuilding=LBuilding-10;
    else
    NLBuilding=0;
    end
    if LProperty>20
    NLProperty=LProperty-20;
    else
    NLProperty=0;
    end
    NLProfit=LProfit;
    NLBC=LBC;
    NL=NLBuilding+NLProperty+NLProfit+NLBC;
  state Init
    Coverage=0;
  state Package3
    Premium=0.06;
    if LBuilding>10
    NLBuilding=LBuilding-10;
    else
    NLBuilding=0;
    end
    if LProfit>35
    NLProfit=LProfit-35;
    else
    NLProfit=0;
    end
    NLProperty=LProperty;
    NLBC=LBC;
    NL=NLBuilding+NLProperty+NLProfit+NLBC;
  state Package5
    Premium=0.005;
    NLBuilding=LBuilding;
    NLProperty=LProperty;
    NLProfit=LProfit
  state Package4
    Premium=0.015;
    if LBuilding>10
    NLBuilding=LBuilding-10;
    else
    NLBuilding=0;
    end
    NLProperty=LProperty;
    NLProfit=LProfit;
  state BC
    if Magnitude>8
    Coverage=7;
    end
    if Magnitude>7
    Coverage=6;
    end
    if Magnitude>6
    Coverage=5;
    end
    if Magnitude>5
    Coverage=4;
    end
    if LBC>Coverage
    NLBC=LBC-Coverage;
    else
    NLBC=0;
    end
    NL=NLBuilding+NLProperty+NLProfit+NLBC;
  Init -> Package1 [order 3] : [Insurance==1&Clock>690]
  Init -> NoInsurance [order 2] : [Insurance==0&Clock>690]
  (default) -> Init
  Init -> Full [order 7] : [Insurance==6&Clock>690]
  Init -> Package2 [order 4] : [Insurance==2&Clock>690]
  Init -> Package5 [order 6] : [Insurance==5&Clock>690]
  Init -> Package3 [order 1] : [Insurance==3&Clock>690]
  Init -> Package4 [order 5] : [Insurance==4&Clock>690]
  Package5 -> BC : [Magnitude>0]
  Package4 -> BC : [Magnitude>0]
  data: LProfit input; LBuilding input; LProperty input; Magnitude input; Insurance input; NL output; Coverage local; Total local; CombinedLoss local; LBC input; Clock input; Premium output; NLBC output; NLBuilding output; NLProfit output; NLProperty output

== stateflow chart Manuf30_M8/Raw Material ==
  state Update
    RawMaterial = RawMaterial + Logistics - Manufacturing
    MxRM=3;
    LxRM=3;
    if RawMaterial < 0
    MxRM=Logistics;
    RawMaterial = 0;
    else if RawMaterial > RMmax
    LxRM=Manufacturing;
    RawMaterial = RMmax;
    end
    end
  state Full
    LxRM=Manufacturing;
    if Logistics >= Manufacturing
    RawMaterial=RMmax;
    else
    RawMaterial = RMmax + Logistics - Manufacturing
    end
  state Init
    RawMaterial=RMdefault;
    MxRM=3;
    LxRM=3;
  state Empty
    MxRM=Logistics;
    if Manufacturing>=Logistics
    RawMaterial=0;
    else
    RawMaterial= Logistics - Manufacturing;
    end
  (default) -> Init
  Update -> Full [order 1] : [RawMaterial>=RMmax]
  Init -> Update : [Manufacturing>0||Logistics>0]
  Full -> Update : [RawMaterial<RMmax]
  Update -> Empty [order 2] : [RawMaterial<=0]
  Empty -> Update : [RawMaterial>0]
  data: Logistics input; RMdefault input; RMmax input; Manufacturing input; MxRM output; LxRM output; RawMaterial output

== stateflow chart Manuf30_M8/Internal ==
  state Init
    IParts=IPdefault;
    MxIP=3;
    AxIP=3;
    DamageIP=0;
  state Update
    MxIP=3;
    AxIP=3;
    if (Inventory<1 && DamageIP==0)
    LossIP=IParts*(1-Inventory);
    IParts=IParts*Inventory;
    DamageIP=1;
    end
    IParts = IParts + Manufacturing - Assembly;
    if IParts < 0
    AxIP=Manufacturing;
    IParts = 0;
    else if IParts > IPmax
    MxIP=Assembly;
    IParts = IPmax;
    end
    end
  state Full
    MxIP=Assembly;
    if Manufacturing >= Assembly
    IParts=IPmax;
    else
    IParts = IPmax + Manufacturing - Assembly
    end
  state Empty
    AxIP=Manufacturing;
    if Assembly>=Manufacturing
    IParts=0;
    else
    IParts= Manufacturing - Assembly;
    end
  (default) -> Init
  Update -> Full [order 1] : [IParts>=IPmax]
  Init -> Update : [Manufacturing>0||Assembly>0||Inventory<1]
  Full -> Update : [IParts<IPmax]
  Update -> Empty [order 2] : [IParts<=0]
  Empty -> Update : [IParts>0]
  data: Assembly input; IPmax input; IPdefault input; Manufacturing input; Inventory input; LossIP output; AxIP output; MxIP output; IParts output; DamageIP local

== stateflow chart Manuf30_M8/State Transition Table9 ==
  state Init
    T=0;
    ITEq=1;
    Damage=0;
  state Great
    ITEq=0;
    RT=30;
    T=T+1;
  state Major
    ITEq=0;
    RT=5;
    T=T+1;
  state Strong
    ITEq=0
    RT=1;
    T=T+1;
  state Moderate
    ITEq=1;
  state ITBackup
    ITEq=0;
    RT=4;
    T=T+1;
  state Over
    ITEq=1;
  (default) -> Init
  Init -> (junction 29) [order 2] : [Magnitude>=7]
      | {Damage=1.5}
  (junction 29) -> (junction 23)
  Init -> (junction 41) [order 3] : [Magnitude>=6]
      | {Damage=0.4}
  (junction 41) -> (junction 39)
  Init -> (junction 44) [order 4] : [Magnitude>=5]
  (junction 44) -> (junction 32)
  Init -> Great [order 1] : [Magnitude>=8]
      | {Damage=2.5}
  Great -> (junction 134) [order 1] : [T>=RT]
  (junction 134) -> (junction 137)
  Great -> (junction 154) [order 2] : [Backup>0]
  (junction 154) -> (junction 157)
  (junction 23) -> Major
  Major -> (junction 137) [order 1] : [T>=RT]
  (junction 137) -> (junction 140)
  Major -> (junction 157) [order 2] : [Backup>0]
  (junction 157) -> (junction 160)
  (junction 39) -> Strong
  Strong -> (junction 140) [order 1] : [T>=RT]
  (junction 140) -> (junction 143)
  Strong -> (junction 160) [order 2] : [Backup>0]
  (junction 160) -> (junction 152)
  (junction 32) -> Moderate
  Moderate -> (junction 143)
  (junction 143) -> (junction 132)
  (junction 152) -> ITBackup
  ITBackup -> Over : [T>=RT]
  (junction 132) -> Over
  data: Magnitude input; T local; RT local; Backup input; ITEq output; Damage output

== stateflow chart Manuf30_M8/State Transition Table ==
  state Normal
    T=0;
    Mnf=0;
  state Level1
    Mnf=0.1;
    T=T+1;
  state Level2
    Mnf=0.22;
    T=T+1;
  state Level3
    Mnf=0.36;
    T=T+1;
  state Level4
    Mnf=0.54;
    T=T+1;
  state Level5
    Mnf=0.74;
    T=T+1;
  state Level6
    Mnf=1;
    T=T+1;
  (default) -> Normal
  (junction 26) -> Normal
  (junction 40) -> (junction 26)
  Normal -> Level1 : [Delayed<=0&Maintenance<=0]
  Level1 -> Normal [order 2] : [Maintenance>0]
  Level1 -> Level2 [order 1] : [Delayed<=0&Maintenance<=0&T>=30]
  Level2 -> (junction 40) [order 2] : [Maintenance>0]
  (junction 46) -> (junction 40)
  Level2 -> Level3 [order 1] : [Delayed<=0&Maintenance<=0&T>=60]
  Level3 -> (junction 46) [order 2] : [Maintenance>0]
  (junction 49) -> (junction 46)
  Level3 -> Level4 [order 1] : [Delayed<=0&Maintenance<=0&T>=90]
  Level4 -> (junction 49) [order 2] : [Maintenance>0]
  (junction 52) -> (junction 49)
  Level4 -> Level5 [order 1] : [Delayed<=0&Maintenance<=0&T>=120]
  Level5 -> (junction 52) [order 2] : [Maintenance>0]
  (junction 56) -> (junction 52)
  Level5 -> Level6 [order 1] : [Delayed<=0&Maintenance<=0&T>=150]
  Level6 -> (junction 56) : [Maintenance>0]
  data: Delayed input; Maintenance input; Mnf output; T local

== stateflow chart Manuf30_M8/Finished Products Warehouse ==
  state Update
    FinishedProducts = FinishedProducts + Assembly - Logistics;
    AxFP=3;
    LxFP=3;
    if FinishedProducts <= 0
    LxFP=Assembly;
    FinishedProducts = 0;
    else if FinishedProducts > FPmax
    AxFP=Logistics;
    FinishedProducts = FPmax;
    end
    end
  state Full
    AxFP=Logistics;
    if Assembly>= Logistics
    FinishedProducts=FPmax;
    else
    FinishedProducts = FPmax + Assembly - Logistics
    end
  state Init
    FinishedProducts=FPdefault;
    AxFP=3;
    LxFP=3;
  state Empty
    LxFP=Assembly;
    if Logistics>=Assembly
    FinishedProducts=0;
    else
    FinishedProducts= Assembly - Logistics;
    end
  (default) -> Init
  Update -> Full [order 1] : [FinishedProducts>=FPmax]
  Init -> Update : [Assembly>0||Logistics>0]
  Full -> Update : [FinishedProducts<FPmax]
  Update -> Empty [order 2] : [FinishedProducts<=0]
  Empty -> Update : [FinishedProducts>0]
  data: FPdefault input; Assembly input; FPmax input; Logistics input; AxFP output; LxFP output; FinishedProducts output

== stateflow chart Manuf30_M8/Chart2 ==
  state RecoveryC
    CR=1;
    if TotalCont-Shipped>Logistics-Contracts
    Level=Logistics;
    else
    Level=TotalCont-Shipped+Contracts;
    Return=1;
    end
    Shipped=Shipped+Level;
    TotalCont=TotalCont+Contracts;
  state Init
    Shipped=0;
    TotalCont=0;
    Level=Logistics*0.5;
    Return=0;
  state Normal
    CR=0;
    Return=0;
    Level=Logistics*0.5;
    Shipped=Shipped+Level;
    TotalCont=TotalCont+Contracts;
  state RecoveryO
    CR=0;
    Level=0.5;
    Shipped=Shipped+Level;
    TotalCont=TotalCont+Contracts;
  (default) -> Init
  Normal -> RecoveryC : [TotalCont>Shipped]
  Init -> Normal : [Level>0]
  RecoveryO -> Normal : [Logistics==1]
  RecoveryC -> RecoveryO : [Return==1]
  data: Logistics input; CR output; TotalCont local; Level output; Shipped local; Contracts input; Return local

== stateflow chart Manuf30_M8/State Transition Table1 ==
  state Init
    T=0;
    MainFacility=1;
    Damage=0;
  state Great
    MainFacility=0;
    RT=120;
    T=T+1;
  state Major
    MainFacility=0;
    RT=60;
    T=T+1;
  state Strong
    MainFacility=0
    RT=3;
    T=T+1;
  state Moderate
    MainFacility=0;
    RT=1;
    T=T+1;
  state Over
    MainFacility=1;
  (default) -> Init
  Init -> (junction 29) [order 3] : [Magnitude>=7]
      | {Damage=3}
  (junction 29) -> (junction 23)
  Init -> (junction 41) [order 4] : [Magnitude>=6]
  (junction 41) -> (junction 39)
  Init -> (junction 151) [order 5] : [Magnitude>=5]
  (junction 151) -> (junction 160)
  Init -> (junction 160) [order 1] : [Magnitude>0 & Reinforcement==1]
  (junction 160) -> (junction 32)
  Init -> Great [order 2] : [Magnitude>=8]
      | {Damage=5}
  Great -> (junction 171) : [T>=RT]
  (junction 171) -> (junction 168)
  (junction 23) -> Major
  Major -> (junction 168) : [T>=RT]
  (junction 168) -> (junction 165)
  (junction 39) -> Strong
  Strong -> (junction 165) : [T>=RT]
  (junction 165) -> (junction 132)
  (junction 32) -> Moderate
  Moderate -> Over : [T>=RT]
  (junction 132) -> Over
  data: Magnitude input; T local; MainFacility output; RT local; Damage output; Reinforcement input

== stateflow chart Manuf30_M8/State Transition Table2 ==
  state Init
    T=0;
    Electricity=1;
  state Great
    Electricity=0;
    RTe=45;
    T=T+1;
  state Major
    Electricity=0;
    RTe=10;
    T=T+1;
  state Strong
    Electricity=0
    RTe=3;
    T=T+1;
  state Moderate
  state Great1
    Electricity=0.4;
    FRe=90;
    T=T+1;
  state Major1
    Electricity=0.5;
    FRe=30;
    T=T+1;
  state Strong1
    Electricity=1;
    FRe=3;
    T=T+1;
  state Over
    Electricity=1;
  (default) -> Init
  Init -> (junction 29) [order 2] : [Magnitude>=7]
  (junction 29) -> (junction 23)
  Init -> (junction 41) [order 3] : [Magnitude>=6]
  (junction 41) -> (junction 39)
  Init -> (junction 44) [order 4] : [Magnitude>=5]
  (junction 44) -> (junction 32)
  Init -> Great [order 1] : [Magnitude>=8]
  Great -> (junction 85) : [T>=RTe]
  (junction 85) -> (junction 83)
  (junction 23) -> Major
  Major -> (junction 112) : [T>=RTe]
  (junction 112) -> (junction 110)
  (junction 39) -> Strong
  Strong -> (junction 123) : [T>=RTe]
  (junction 123) -> (junction 121)
  (junction 32) -> Moderate
  (junction 83) -> Great1
  Great1 -> (junction 107) : [T>=FRe]
  (junction 107) -> (junction 117)
  (junction 110) -> Major1
  Major1 -> (junction 117) : [T>=FRe]
  (junction 117) -> (junction 105)
  (junction 121) -> Strong1
  Strong1 -> Over : [T>=FRe]
  (junction 105) -> Over
  data: Magnitude input; T local; Electricity output; RTe local; FRe local

== stateflow chart Manuf30_M8/State Transition Table3 ==
  state Init
    T=0;
    Maintenance=1;
  state Great
    Maintenance=0;
    RTm=120;
    T=T+1;
  state Major
    Maintenance=0;
    RTm=45;
    T=T+1;
  state Strong
    Maintenance=0
    RTm=10;
    T=T+1;
  state Moderate
  state Great1
    Maintenance=1;
    FRm=120;
    T=T+1;
  state Major1
    Maintenance=1;
    FRm=45;
    T=T+1;
  state Strong1
    Maintenance=1;
    FRm=10;
    T=T+1;
  state Over
    Maintenance=1;
  (default) -> Init
  Init -> (junction 29) [order 2] : [Magnitude>=7]
  (junction 29) -> (junction 23)
  Init -> (junction 41) [order 3] : [Magnitude>=6]
  (junction 41) -> (junction 39)
  Init -> (junction 44) [order 4] : [Magnitude>=5]
  (junction 44) -> (junction 32)
  Init -> Great [order 1] : [Magnitude>=8]
  Great -> (junction 85) : [T>=RTm]
  (junction 85) -> (junction 83)
  (junction 23) -> Major
  Major -> (junction 112) : [T>=RTm]
  (junction 112) -> (junction 110)
  (junction 39) -> Strong
  Strong -> (junction 123) : [T>=RTm]
  (junction 123) -> (junction 121)
  (junction 32) -> Moderate
  (junction 83) -> Great1
  Great1 -> (junction 107) : [T>=FRm]
  (junction 107) -> (junction 117)
  (junction 110) -> Major1
  Major1 -> (junction 117) : [T>=FRm]
  (junction 117) -> (junction 105)
  (junction 121) -> Strong1
  Strong1 -> Over : [T>=FRm]
  (junction 105) -> Over
  data: Magnitude input; T local; RTm local; FRm local; Maintenance output

== stateflow chart Manuf30_M8/State Transition Table4 ==
  state Init
    T=0;
    Logistics=1;
  state Great
    Logistics=0;
    RTl=75;
    T=T+1;
  state Major
    Logistics=0;
    RTl=30;
    T=T+1;
  state Strong
    Logistics=0
    RTl=3;
    T=T+1;
  state Moderate
  state Great1
    Logistics=0.3;
    FRl=145;
    T=T+1;
  state Major1
    Logistics=0.5;
    FRl=60;
    T=T+1;
  state Strong1
    Logistics=1;
    FRl=3;
    T=T+1;
  state Over
    Logistics=1;
  (default) -> Init
  Init -> (junction 29) [order 2] : [Magnitude>=7]
  (junction 29) -> (junction 23)
  Init -> (junction 41) [order 3] : [Magnitude>=6]
  (junction 41) -> (junction 39)
  Init -> (junction 44) [order 4] : [Magnitude>=5]
  (junction 44) -> (junction 32)
  Init -> Great [order 1] : [Magnitude>=8]
  Great -> (junction 85) : [T>=RTl]
  (junction 85) -> (junction 83)
  (junction 23) -> Major
  Major -> (junction 112) : [T>=RTl]
  (junction 112) -> (junction 110)
  (junction 39) -> Strong
  Strong -> (junction 123) : [T>=RTl]
  (junction 123) -> (junction 121)
  (junction 32) -> Moderate
  (junction 83) -> Great1
  Great1 -> (junction 107) : [T>=FRl]
  (junction 107) -> (junction 117)
  (junction 110) -> Major1
  Major1 -> (junction 117) : [T>=FRl]
  (junction 117) -> (junction 105)
  (junction 121) -> Strong1
  Strong1 -> Over : [T>=FRl]
  (junction 105) -> Over
  data: Magnitude input; T local; RTl local; FRl local; Logistics output
